simulink model "task_B_mod"  (R2018a)
settings: Solver=ode45  StartTime=0.0  StopTime=10.0  RelTol=1e-3  EnableMultiTasking=on
values from neighbouring files (symbols this model uses):
  A = [0,1;-c/m,-beta/m]    [task_A_scr.m]    (also in task_B_scr.m = A*(16*lamda/(c*ro*h^2)); task_C1_scr.m = A*(16*lamda/(c*ro*h^2)); task_C_scr.m = A*(16*lamda/(c*ro*h^2)); task_D1_scr.m = A*(16*lamda/(c*ro*h^2)))
  B = [0;1]    [task_A_scr.m]    (also in task_B_scr.m = B*(4/(c*ro*h)); task_C1_scr.m = B*(4/(c*ro*h)); task_C_scr.m = B*(4/(c*ro*h)); task_D1_scr.m = B*(4/(c*ro*h)))
  qa = 500000    [task_B_scr.m]    (also in task_C1_scr.m = 650000; task_C_scr.m; task_D1_scr.m = 550000; task_D2_scr.m)
  T_0 = 300    [task_B_scr.m]    (also in task_C1_scr.m; task_C_scr.m; task_D1_scr.m; task_D2_scr.m)
  Tb = 350    [task_B_scr.m]    (also in task_C1_scr.m = 403; sim('task_C1_mod',15); task_C_scr.m; task_D1_scr.m; task_D2_scr.m = 350; sim('task_D1_mod',10))
settings Model: Creator=Yurii  LastModifiedBy=Master
settings DataIOCC: LimitDataPoints=on  SaveFormat=Array
settings OptimizationCC: LifeSpan=inf
settings DebuggingCC: UnderspecifiedInitializationDetection=Classic  MergeDetectMultiDrivingBlocksExec=none  SolverPrmCheckMsg=warning  SFUnexpectedBacktrackingDiag=warning  SFNoUnconditionalDefaultTransitionDiag=warning  SFExecutionAtInitializationDiag=none
settings HardwareCC: ProdBitPerPointer=32  ProdBitPerSizeT=32  ProdBitPerPtrDiffT=32  ProdLargestAtomicFloat=None  ProdIntDivRoundTo=Undefined  ProdEndianess=Unspecified  ProdWordSize=32  ProdHWDeviceType=32-bit Generic
settings ModelReferenceCC: PropagateSignalLabelsOutOfModel=off
settings CodeAppCC: StateflowObjectComments=on
settings GRTTargetCC: TargetLangStandard=C89/C90 (ANSI)  GeneratePreprocessorConditionals=Disable all
settings ConfigComp: CovMetricSettings=dw  CovHtmlReporting=on  CovSaveCumulativeToWorkspaceVar=on  CovSaveSingleToWorkspaceVar=on  CovExternalEMLEnable=off

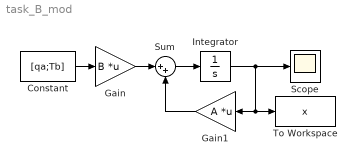
== system task_B_mod ==
  Constant : Constant  Value=[qa;Tb]
  Gain : Gain  Gain=B  Multiplication=Matrix(K*u)
  Gain1 : Gain  Gain=A  Multiplication=Matrix(K*u)
  Integrator : Integrator  InitialCondition=[T_0;T_0;T_0]
  Scope : Scope
  Sum : Sum  Inputs=|++
  To Workspace : ToWorkspace  VariableName=x  SaveFormat=Timeseries  SampleTime=-1
  wires:
  Constant/1 -> Gain/1
  Gain/1 -> Sum/1
  Sum/1 -> Integrator/1
  Gain1/1 -> Sum/2
  Integrator/1 -> Gain1/1, To Workspace/1, Scope/1
